simulink model "Bebop8_KF_filter"  (R2018a)
settings: Solver=VariableStepAuto  StartTime=0.0  StopTime=50  FixedStep=.04  MaxStep=1.00  MinStep=0.005  RelTol=10  AbsTol=10
values from neighbouring files (symbols this model uses):
  flightplan = [dist,0,height,deg2rad(090) ... (first row only)    [compare_cubic_spline_1.m]    (also in initialize_race_realtime.m = [dist+1,0,height,deg2rad(090); initialize_race_realtime_backup_cubic.m; plot_sim.m = [ 4.348, -0.278, height, deg2rad(  0); test_b_spline.m)
  FOV = 1.05    [initialize_race_realtime.m]    (also in initialize_race_realtime_backup_cubic.m)
  g = 9.81    [initialize_race_no_realtime.m]    (also in initialize_race_realtime.m; initialize_race_realtime_backup_cubic.m; moving_average_rls_own.m = P(i-1)*meas*(lambda+meas*P(i-1)*meas)^-1)
  gate_size = 1.4    [initialize_race_realtime.m]    (also in initialize_race_realtime_backup_cubic.m)
  gates = sim_gates(:,:,1)    [eval_sim.m]    (also in initialize_race_realtime.m = [dist+1,0,height,deg2rad(110); initialize_race_realtime_backup_cubic.m = [dist,0,height,deg2rad(110); plot_sim.m)
  I = [1 0 0 ... (first row only)    [Bebop_sim_init.m]    (also in initialize_race_no_realtime.m; initialize_race_realtime.m; initialize_race_realtime_backup_cubic.m; moving_averge_rls_download.m = ones(1,N))
  init_std_dev = [1.0*ones(1,3),deg2rad(30)]    [initialize_race_realtime.m]    (also in initialize_race_realtime_backup_cubic.m)
  m = 0.68    [calc_plot_spline.m]    (also in calc_spline.m; compare_cubic_spline_1.m = vpasolve(e,r); compare_cubic_spline_2.m = r/3*(-sin(dp)+sqrt(sin(dp)^2-6*cos(dp)+6)); initialize_race_no_realtime.m = 2)
  max_rot_Z = (90)*pi/180    (= 1.57079632679)    [Bebop_sim_init.m]    (also in initialize_race_no_realtime.m = 1.0471975512; initialize_race_realtime.m = 1.0471975512; initialize_race_realtime_backup_cubic.m; run_batch1.m = list_agility(idx_agility)*max_rot_Z)
  max_theta_X = (40)*pi/180    (= 0.698131700798)    [Bebop_sim_init.m]    (also in initialize_race_no_realtime.m = 0.13962634016; initialize_race_realtime.m = 1.308996939; initialize_race_realtime_backup_cubic.m = 1.308996939; run_batch1.m = list_agility(idx_agility)*max_theta_X)
  max_theta_Y = (40)*pi/180    (= 0.698131700798)    [Bebop_sim_init.m]    (also in initialize_race_no_realtime.m = 0.13962634016; initialize_race_realtime.m = 1.308996939; initialize_race_realtime_backup_cubic.m = 1.308996939; run_batch1.m = list_agility(idx_agility)*max_theta_Y)
  max_v_Z = .5    (= 0.5)    [Bebop_sim_init.m]    (also in initialize_race_no_realtime.m = 1; initialize_race_realtime.m = 2; initialize_race_realtime_backup_cubic.m = 3; run_batch1.m = list_agility(idx_agility)*max_v_Z)
  max_vel = 1.0    (= 1)    [initialize_race_realtime.m]    (also in initialize_race_realtime_backup_cubic.m = 1.5; run_batch1.m = list_speed(idx_speed); run_batch2.m = list_speed(idx_speed); run_batch3.m = list_speed(idx_speed))
  spline_init = [P0;P1;P2;P3]    [initialize_race_realtime.m]
  std_dev_factor = 1.0    (= 1)    [initialize_race_realtime.m]
  std_dev_switch = std_dev_factor/5    (= 0.2)    [initialize_race_realtime.m]
undefined symbols (not defined in the file or in its folder): fspecial, gray, Rec, SDTV
libraries: simulink x11, sharedtransform x11, visiontextngfix x7, visionanalysis x7, visiontransforms x3, aerolibactuator x2, aerolibutil x2, visionstatistics x2, visionconversions x2, shared6dof x1, vrlib x1, visionsinks x1
(part 3 of 4)

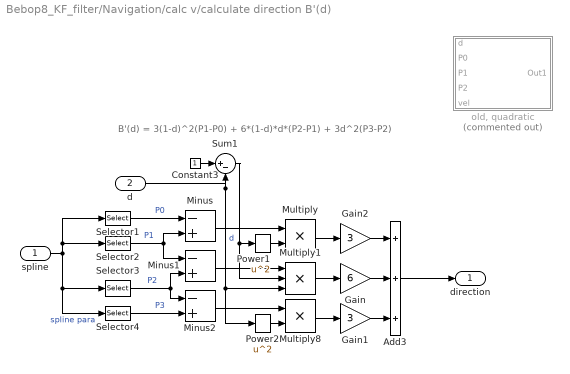
== system Bebop8_KF_filter/Navigation/calc v/calculate direction B'(d) ==
  note: B'(d) = 3(1-d)^2(P1-P0) + 6*(1-d)*d*(P2-P1) + 3d^2(P3-P2)
  spline : Inport
  d : Inport  Port=2
  Add3 : Sum  Inputs=+++
  Constant3 : Constant
  Gain : Gain  Gain=6
  Gain1 : Gain  Gain=3
  Gain2 : Gain  Gain=3
  Minus : Sum  Inputs=-+
  Minus1 : Sum  Inputs=-+
  Minus2 : Sum  Inputs=-+
  Multiply : Product
  Multiply1 : Product  Inputs=3
  Multiply8 : Product
  Power1 : Math  Operator=square  SaturateOnIntegerOverflow=on
  Power2 : Math  Operator=square  SaturateOnIntegerOverflow=on
  Selector1 : Selector  NumberOfDimensions=2  IndexMode=Zero-based  InputPortWidth=3  IndexOptions=Index vector (dialog),Select all  Indices=0,[0 1 2]  OutputSizes=1,1
  Selector2 : Selector  NumberOfDimensions=2  IndexMode=Zero-based  InputPortWidth=3  IndexOptions=Index vector (dialog),Select all  Indices=1,[0 1 2]  OutputSizes=1,1
  Selector3 : Selector  NumberOfDimensions=2  IndexMode=Zero-based  InputPortWidth=3  IndexOptions=Index vector (dialog),Select all  Indices=2,[0 1 2]  OutputSizes=1,1
  Selector4 : Selector  NumberOfDimensions=2  IndexMode=Zero-based  InputPortWidth=3  IndexOptions=Index vector (dialog),Select all  Indices=3,[0 1 2]  OutputSizes=1,1
  Sum1 : Sum  Inputs=|+-
  "old, quadratic" : Subsystem  Commented=on
  direction : Outport
  wires:
  Sum1/1 -> Multiply1/2, Power1/1
  Minus1/1 -> Multiply1/1
  Minus/1 -> Multiply/1
  Gain/1 -> Add3/2
  Gain1/1 -> Add3/3
  Multiply1/1 -> Gain/1
  Minus2/1 -> Multiply8/1
  Constant3/1 -> Sum1/1
  Multiply/1 -> Gain2/1
  Multiply8/1 -> Gain1/1
  Power2/1 -> Multiply8/2
  Power1/1 -> Multiply/2
  d/1 -> Sum1/2, Power2/1, Multiply1/3  "d"
  Gain2/1 -> Add3/1
  Add3/1 -> direction/1
  Selector1/1 -> Minus/1  "P0"
  Selector3/1 -> Minus2/1, Minus1/2  "P2"
  spline/1 -> Selector2/1, Selector1/1, Selector4/1, Selector3/1  "spline para"
  Selector2/1 -> Minus1/1, Minus/2  "P1"
  Selector4/1 -> Minus2/2  "P3"

== system Bebop8_KF_filter/Navigation/calc v/min spd ==
  In1 : Inport
  Abs : Abs
  Add : Sum  Inputs=+-
  Constant : Constant  Value=0.01
  Constant1 : Constant  Value=0.5
  Minus : Sum  Inputs=+-
  Multiply : Product
  Saturation : Saturate  UpperLimit=0  LowerLimit=-1
  Scope : Scope  NumInputPorts=7
  Sign : Signum
  Sign1 : Signum
  Sum : Sum  Inputs=|++
  Out1 : Outport
  wires:
  In1/1 -> Scope/1, Add/1, Sign/1, Abs/1
  Abs/1 -> Minus/1
  Constant/1 -> Minus/2
  Minus/1 -> Scope/4, Saturation/1
  Saturation/1 -> Scope/5, Multiply/1
  Sum/1 -> Sign1/1
  Multiply/1 -> Scope/2, Add/2
  Add/1 -> Scope/3, Out1/1
  Constant1/1 -> Sum/2
  Sign1/1 -> Multiply/2
  Sign/1 -> Sum/1

== system Bebop8_KF_filter/Navigation/calculate desired/If Action Subsystem ==
  In1 : Inport
  Action Port : ActionPort  ActionType=then
  Out1 : Outport
  wires:
  In1/1 -> Out1/1

== system Bebop8_KF_filter/Navigation/calculate desired/If Action Subsystem1 ==
  In1 : Inport
  Action Port : ActionPort  ActionType=else
  Out1 : Outport
  wires:
  In1/1 -> Out1/1

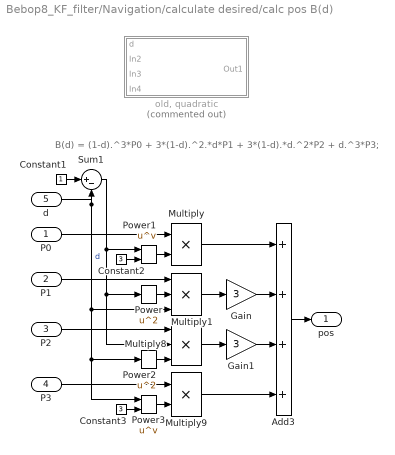
== system Bebop8_KF_filter/Navigation/calculate desired/calc pos B(d) ==
  note: B(d) = (1-d).^3*P0 + 3*(1-d).^2.*d*P1 + 3*(1-d).*d.^2*P2 + d.^3*P3;
  P0 : Inport
  P1 : Inport  Port=2
  P2 : Inport  Port=3
  P3 : Inport  Port=4
  d : Inport  Port=5
  Add3 : Sum  Inputs=++++
  Constant1 : Constant
  Constant2 : Constant  Value=3
  Constant3 : Constant  Value=3
  Gain : Gain  Gain=3
  Gain1 : Gain  Gain=3
  Multiply : Product
  Multiply1 : Product  Inputs=3
  Multiply8 : Product  Inputs=3
  Multiply9 : Product
  Power : Math  Operator=square  SaturateOnIntegerOverflow=on
  Power1 : Math  Operator=pow  SaturateOnIntegerOverflow=on
  Power2 : Math  Operator=square  SaturateOnIntegerOverflow=on
  Power3 : Math  Operator=pow  SaturateOnIntegerOverflow=on
  Sum1 : Sum  Inputs=|+-
  "old, quadratic" : Subsystem  Commented=on
  pos : Outport
  wires:
  Gain/1 -> Add3/2
  Gain1/1 -> Add3/3
  P1/1 -> Multiply1/1
  P0/1 -> Multiply/1
  P2/1 -> Multiply8/1
  P3/1 -> Multiply9/1
  Multiply/1 -> Add3/1
  Multiply1/1 -> Gain/1
  Multiply8/1 -> Gain1/1
  Multiply9/1 -> Add3/4
  Add3/1 -> pos/1
  Constant1/1 -> Sum1/1
  d/1 -> Sum1/2, Multiply1/3, Power2/1, Power3/1  "d"
  Power/1 -> Multiply1/2
  Power1/1 -> Multiply/2
  Power2/1 -> Multiply8/3
  Power3/1 -> Multiply9/2
  Constant2/1 -> Power1/2
  Constant3/1 -> Power3/2
  Sum1/1 -> Multiply8/2, Power/1, Power1/1

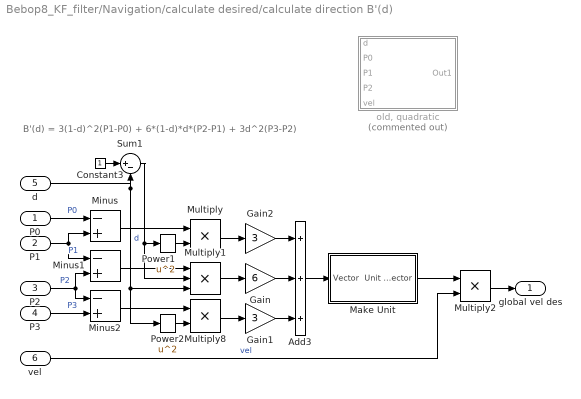
== system Bebop8_KF_filter/Navigation/calculate desired/calculate direction B'(d) ==
  note: B'(d) = 3(1-d)^2(P1-P0) + 6*(1-d)*d*(P2-P1) + 3d^2(P3-P2)
  P0 : Inport
  P1 : Inport  Port=2
  P2 : Inport  Port=3
  P3 : Inport  Port=4
  d : Inport  Port=5
  vel : Inport  Port=6
  Add3 : Sum  Inputs=+++
  Constant3 : Constant
  Gain : Gain  Gain=6
  Gain1 : Gain  Gain=3
  Gain2 : Gain  Gain=3
  Make Unit : Subsystem
  Minus : Sum  Inputs=-+
  Minus1 : Sum  Inputs=-+
  Minus2 : Sum  Inputs=-+
  Multiply : Product
  Multiply1 : Product  Inputs=3
  Multiply2 : Product
  Multiply8 : Product
  Power1 : Math  Operator=square  SaturateOnIntegerOverflow=on
  Power2 : Math  Operator=square  SaturateOnIntegerOverflow=on
  Sum1 : Sum  Inputs=|+-
  "old, quadratic" : Subsystem  Commented=on
  global vel des : Outport
  wires:
  Sum1/1 -> Multiply1/2, Power1/1
  Minus1/1 -> Multiply1/1
  Minus/1 -> Multiply/1
  Gain/1 -> Add3/2
  Gain1/1 -> Add3/3
  Multiply1/1 -> Gain/1
  Minus2/1 -> Multiply8/1
  Constant3/1 -> Sum1/1
  Multiply/1 -> Gain2/1
  Multiply8/1 -> Gain1/1
  Power2/1 -> Multiply8/2
  Power1/1 -> Multiply/2
  d/1 -> Sum1/2, Power2/1, Multiply1/3  "d"
  Gain2/1 -> Add3/1
  P0/1 -> Minus/1  "P0"
  P1/1 -> Minus/2, Minus1/1  "P1"
  P2/1 -> Minus1/2, Minus2/1  "P2"
  P3/1 -> Minus2/2  "P3"
  Multiply2/1 -> global vel des/1
  Add3/1 -> Make Unit/1(Vector)
  Make Unit/1(Unit Vector) -> Multiply2/1
  vel/1 -> Multiply2/2  "vel"

== system Bebop8_KF_filter/Navigation/calculate desired/min gate distance ==
  Constant2 : Constant  Value=gate_size
  Constant3 : Constant  Value=FOV
  Divide : Product  Inputs=*/
  Gain1 : Gain  Gain=0.5
  Gain2 : Gain  Gain=0.5
  Tan : Trigonometry  Operator=tan
  min gate dist : Outport
  wires:
  Constant3/1 -> Gain2/1
  Constant2/1 -> Gain1/1
  Gain1/1 -> Divide/1
  Gain2/1 -> Tan/1
  Divide/1 -> min gate dist/1  "min dist"
  Tan/1 -> Divide/2

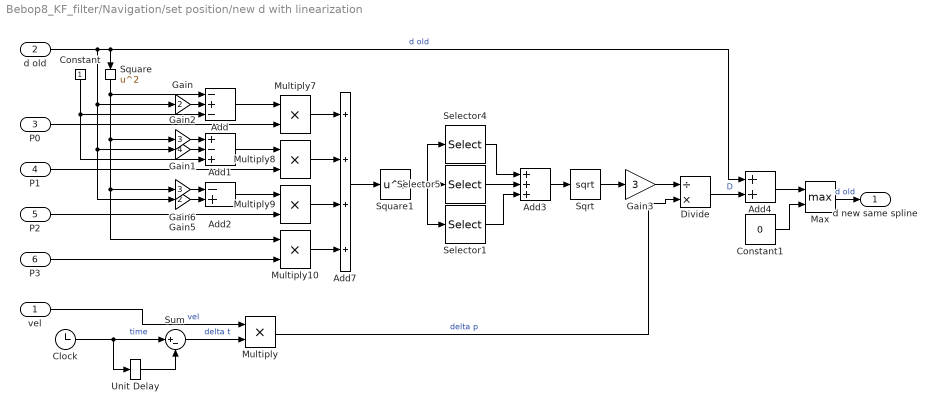
== system Bebop8_KF_filter/Navigation/set position/new d with linearization ==
  vel : Inport
  d old : Inport  Port=2
  P0 : Inport  Port=3
  P1 : Inport  Port=4
  P2 : Inport  Port=5
  P3 : Inport  Port=6
  Add : Sum  Inputs=-+-
  Add1 : Sum  Inputs=+-+
  Add2 : Sum  Inputs=-+
  Add3 : Sum  Inputs=+++
  Add4 : Sum
  Add7 : Sum  Inputs=++++
  Clock : Clock
  Constant : Constant
  Constant1 : Constant  Value=0
  Divide : Product  Inputs=/*
  Gain : Gain  Gain=2
  Gain1 : Gain  Gain=4
  Gain2 : Gain  Gain=3
  Gain3 : Gain  Gain=3
  Gain5 : Gain  Gain=2
  Gain6 : Gain  Gain=3
  Max : MinMax  Function=max  Inputs=2
  Multiply{,7..10} (5 alike) : Product
  Selector1 : Selector  IndexMode=Zero-based  InputPortWidth=3  IndexOptions=Index vector (dialog)  Indices=2  OutputSizes=1
  Selector4 : Selector  IndexMode=Zero-based  InputPortWidth=3  IndexOptions=Index vector (dialog)  Indices=0  OutputSizes=1
  Selector5 : Selector  IndexMode=Zero-based  InputPortWidth=3  IndexOptions=Index vector (dialog)  Indices=1  OutputSizes=1
  Sqrt : Sqrt  SaturateOnIntegerOverflow=on
  Square : Math  Operator=square  SaturateOnIntegerOverflow=on
  Square1 : Math  Operator=square  SaturateOnIntegerOverflow=on
  Sum : Sum  Inputs=|+-
  Unit Delay : UnitDelay  SampleTime=-1
  d new same spline : Outport
  wires:
  Add7/1 -> Square1/1
  Multiply8/1 -> Add7/2
  Multiply9/1 -> Add7/3
  Square/1 -> Multiply10/1, Gain6/1, Gain2/1, Add/1
  Gain/1 -> Add/2
  Constant/1 -> Add1/3, Add/3
  Gain2/1 -> Add1/1
  Gain1/1 -> Add1/2
  Gain6/1 -> Add2/1
  Gain5/1 -> Add2/2
  Multiply10/1 -> Add7/4
  Add2/1 -> Multiply9/1
  Add1/1 -> Multiply8/1
  Add/1 -> Multiply7/1
  Multiply7/1 -> Add7/1
  Selector5/1 -> Add3/2
  Multiply/1 -> Divide/2  "delta p"
  Gain3/1 -> Divide/1
  Divide/1 -> Add4/2  "D"
  Selector4/1 -> Add3/1
  Add3/1 -> Sqrt/1
  Square1/1 -> Selector1/1, Selector4/1, Selector5/1
  Sqrt/1 -> Gain3/1
  Selector1/1 -> Add3/3
  Sum/1 -> Multiply/2  "delta t"
  Unit Delay/1 -> Sum/2
  vel/1 -> Multiply/1  "vel"
  Clock/1 -> Unit Delay/1, Sum/1  "time"
  Add4/1 -> Max/1
  Constant1/1 -> Max/2
  P1/1 -> Multiply8/2
  P2/1 -> Multiply9/2
  P0/1 -> Multiply7/2
  Max/1 -> d new same spline/1  "d old"
  P3/1 -> Multiply10/2
  d old/1 -> Add4/1, Square/1, Gain/1, Gain5/1, Gain1/1  "d old"

== system Bebop8_KF_filter/Vision System/Harris corner detection/Harris Corners ==
  Threshold : Inport
  Corner Detection : visionanalysis/Corner Detection  method=Harris corner detection (Harris & Stephens)  factor=0.01  filter=fspecial('gaussian', [1 9], 3)  thrInten=0.1  thrAngle=157.5  output=Obsolete9b  outputInUse=Corner location  maxNum=5  thrMetric=0.01  neighborSize=[25 25]  isOutVarDim=on  accumMode=Binary point scaling  accumWordLength=32  accumFracLength=0  prodOutputMode=Binary point scaling  prodOutputWordLength=32  prodOutputFracLength=0  memoryMode=Binary point scaling  memoryWordLength=32  memoryFracLength=0  firstCoeffMode=Specify word length  firstCoeffWordLength=16  firstCoeffFracLength=17  roundingMode=Floor  overflowMode=off
      settings: SourceProductName=Computer Vision System Toolbox  SourceProductBaseCode=VP
  Gaussian Pyramid : visiontransforms/Gaussian Pyramid  Commented=on  operation=Expand  level=1  source=Specify via dialog  a=0.375  coef=fspecial('gaussian', [1 9], 3)  hiddenCoef=fspecial('gaussian', [1 9], 3)  firstCoeffMode=Specify word length  firstCoeffWordLength=16  firstCoeffFracLength=17  outputMode=Binary point scaling  outputWordLength=32  outputFracLength=10  prodOutputMode=Binary point scaling  prodOutputWordLength=32  prodOutputFracLength=10  roundingMode=Floor  overflowMode=off
      settings: SourceProductName=Computer Vision System Toolbox  SourceProductBaseCode=VP
  Video Viewer2 : VideoViewer  Commented=on  colormapValue=gray(256)  FigPos=[76 898 768 763]
  Corners : Outport
  wires:
  Threshold/1 -> Gaussian Pyramid/1, Corner Detection/1
  Gaussian Pyramid/1 -> Video Viewer2/1
  Corner Detection/1 -> Corners/1

== system Bebop8_KF_filter/Vision System/Harris corner detection/calculate corners ==
  In1 : Inport
  Action Port : ActionPort  PropagateVarSize=During execution  ActionType=then
  calculate corners : MATLAB Function  TreatAsAtomicUnit=on
  Out1 : Outport
  wires:
  In1/1 -> calculate corners/1(corners)
  calculate corners/1(corners_four) -> Out1/1

== system Bebop8_KF_filter/Control/Create Path Frame/Make X Vector/Make Unit ==
  Vector : Inport
  Multiply : Product
  Reciprocal Sqrt : Sqrt  Operator=rSqrt  SaturateOnIntegerOverflow=on
  Square : Math  Operator=square  SaturateOnIntegerOverflow=on
  Sum of Elements : Sum  Inputs=+
  Unit Vector : Outport
  wires:
  Reciprocal Sqrt/1 -> Multiply/1
  Vector/1 -> Square/1, Multiply/2
  Square/1 -> Sum of Elements/1
  Multiply/1 -> Unit Vector/1
  Sum of Elements/1 -> Reciprocal Sqrt/1

== system Bebop8_KF_filter/Control/Create Path Frame/Make Y Vector/Make Unit ==
  Vector : Inport
  Multiply : Product
  Reciprocal Sqrt : Sqrt  Operator=rSqrt  SaturateOnIntegerOverflow=on
  Square : Math  Operator=square  SaturateOnIntegerOverflow=on
  Sum of Elements : Sum  Inputs=+
  Unit Vector : Outport
  wires:
  Reciprocal Sqrt/1 -> Multiply/1
  Vector/1 -> Square/1, Multiply/2
  Square/1 -> Sum of Elements/1
  Multiply/1 -> Unit Vector/1
  Sum of Elements/1 -> Reciprocal Sqrt/1

== system Bebop8_KF_filter/Control/Create Path Frame/Make Z Vector/Make Unit ==
  Vector : Inport
  Multiply : Product
  Reciprocal Sqrt : Sqrt  Operator=rSqrt  SaturateOnIntegerOverflow=on
  Square : Math  Operator=square  SaturateOnIntegerOverflow=on
  Sum of Elements : Sum  Inputs=+
  Unit Vector : Outport
  wires:
  Reciprocal Sqrt/1 -> Multiply/1
  Vector/1 -> Square/1, Multiply/2
  Square/1 -> Sum of Elements/1
  Multiply/1 -> Unit Vector/1
  Sum of Elements/1 -> Reciprocal Sqrt/1

== system Bebop8_KF_filter/Navigation/calc v/Create Path Frame/Make X Vector ==
  Velocity Vector : Inport
  Make Unit : Subsystem
  Transpose : Math  Operator=transpose  SaturateOnIntegerOverflow=on
  X Vector : Outport
  wires:
  Velocity Vector/1 -> Make Unit/1(Vector)
  Make Unit/1(Unit Vector) -> Transpose/1
  Transpose/1 -> X Vector/1

== system Bebop8_KF_filter/Navigation/calc v/Create Path Frame/Make Y Vector ==
  Velocity Vector : Inport
  Constant : Constant  Value=0
  Demux : Demux  Outputs=3
  Gain : Gain  Gain=-1
  Make Unit : Subsystem
  Matrix Concatenate : Concatenate  NumInputs=3  Mode=Multidimensional array
  Terminator : Terminator
  Y Vector : Outport
  wires:
  Make Unit/1(Unit Vector) -> Y Vector/1
  Velocity Vector/1 -> Demux/1
  Demux/3 -> Terminator/1
  Demux/2 -> Gain/1
  Gain/1 -> Matrix Concatenate/1
  Demux/1 -> Matrix Concatenate/2
  Constant/1 -> Matrix Concatenate/3
  Matrix Concatenate/1 -> Make Unit/1(Vector)

== system Bebop8_KF_filter/Navigation/calc v/Create Path Frame/Make Z Vector ==
  Velocity Vector : Inport
  Add : Sum
  Demux : Demux  Outputs=3
  Gain : Gain  Gain=-1
  Gain1 : Gain  Gain=-1
  Make Unit : Subsystem
  Matrix Concatenate : Concatenate  NumInputs=3  Mode=Multidimensional array
  Multiply : Product
  Multiply1 : Product
  Square : Math  Operator=square  SaturateOnIntegerOverflow=on
  Square1 : Math  Operator=square  SaturateOnIntegerOverflow=on
  Z Vector : Outport
  wires:
  Make Unit/1(Unit Vector) -> Z Vector/1
  Velocity Vector/1 -> Demux/1
  Demux/3 -> Multiply/2, Multiply1/2
  Matrix Concatenate/1 -> Make Unit/1(Vector)
  Multiply/1 -> Gain/1
  Gain/1 -> Matrix Concatenate/1
  Demux/1 -> Square/1, Multiply/1
  Multiply1/1 -> Gain1/1
  Gain1/1 -> Matrix Concatenate/2
  Demux/2 -> Square1/1, Multiply1/1
  Add/1 -> Matrix Concatenate/3
  Square/1 -> Add/1
  Square1/1 -> Add/2

== system Bebop8_KF_filter/Navigation/calc v/calculate direction B'(d)/old, quadratic ==
  note: B'(d) = 2(1-d)(P1-P0) + 2d(P2-P1) = 2*(dP0-2dP1+dP2+P1-P0)
  d : Inport
  P0 : Inport  Port=2
  P1 : Inport  Port=3
  P2 : Inport  Port=4
  vel : Inport  Port=5
  Add1 : Sum  Commented=on  Inputs=+--++-
  Atan1 : Trigonometry  Commented=on  Operator=atan2
  Constant1 : Constant  Commented=on  Value=0
  Constant2 : Constant  Commented=on  Value=0
  Matrix Multiply : Product  Commented=on  Inputs=/*  Multiplication=Matrix(*)
  Product : Product  Commented=on
  Product1 : Product  Commented=on
  Product2 : Product  Commented=on
  Rotation Angles to Direction Cosine Matrix1 : sharedtransform/Rotation Angles to Direction Cosine Matrix  Commented=on  rotationOrder=ZYX  aMode=aMode
      settings: SourceProductBaseCode=AE
  Selector7 : Selector  Commented=on  IndexMode=Zero-based  InputPortWidth=3  IndexOptions=Index vector (dialog)  Indices=1  OutputSizes=1
  Selector8 : Selector  Commented=on  IndexMode=Zero-based  InputPortWidth=3  IndexOptions=Index vector (dialog)  Indices=0  OutputSizes=1
  Vector Concatenate : Concatenate  Commented=on  NumInputs=3
  Vector Concatenate1 : Concatenate  Commented=on  NumInputs=3
  Out1 : Outport
  wires:
  Product2/1 -> Add1/4
  P1/1 -> Add1/5, Product1/2
  Rotation Angles to Direction Cosine Matrix1/1 -> Matrix Multiply/1  "rot matrix"
  P2/1 -> Product2/2
  Add1/1 -> Selector8/1, Selector7/1
  Product/1 -> Add1/1
  P0/1 -> Add1/6, Product/2
  d/1 -> Product2/1, Product1/1, Product/1
  Constant1/1 -> Vector Concatenate/2, Vector Concatenate/3
  Vector Concatenate1/1 -> Matrix Multiply/2
  Product1/1 -> Add1/3, Add1/2
  Vector Concatenate/1 -> Rotation Angles to Direction Cosine Matrix1/1
  Selector7/1 -> Atan1/1
  vel/1 -> Vector Concatenate1/1
  Constant2/1 -> Vector Concatenate1/2, Vector Concatenate1/3
  Matrix Multiply/1 -> Out1/1
  Selector8/1 -> Atan1/2
  Atan1/1 -> Vector Concatenate/1  "yaw"

== system Bebop8_KF_filter/Navigation/calculate desired/calc pos B(d)/old, quadratic ==
  note: B(d) = (1-d)*u.*((1-d)*P0+d*P1)+d*u.*((1-d)*P1 + d*P2);
  d : Inport
  In2 : Inport  Port=2
  In3 : Inport  Port=3
  In4 : Inport  Port=4
  Add : Sum  Commented=on
  Add1 : Sum  Commented=on
  Add2 : Sum  Commented=on
  Constant : Constant  Commented=on
  Multiply{2..7} (6 alike) : Product  Commented=on
  Sum : Sum  Commented=on  Inputs=|+-
  Out1 : Outport
  wires:
  In4/1 -> Multiply5/1
  Constant/1 -> Sum/1
  Multiply7/1 -> Add2/2
  d/1 -> Multiply5/2, Multiply7/1, Multiply3/1, Sum/2
  Multiply3/1 -> Add/2
  Multiply5/1 -> Add1/2
  Multiply4/1 -> Add1/1
  Sum/1 -> Multiply4/2, Multiply6/2, Multiply2/1  "1-d"
  In3/1 -> Multiply4/1, Multiply3/2
  Multiply2/1 -> Add/1
  Add2/1 -> Out1/1
  Add1/1 -> Multiply7/2
  Multiply6/1 -> Add2/1
  In2/1 -> Multiply2/2
  Add/1 -> Multiply6/1

== system Bebop8_KF_filter/Navigation/calculate desired/calculate direction B'(d)/Make Unit ==
  Vector : Inport
  Multiply : Product
  Reciprocal Sqrt : Sqrt  Operator=rSqrt  SaturateOnIntegerOverflow=on
  Square : Math  Operator=square  SaturateOnIntegerOverflow=on
  Sum of Elements : Sum  Inputs=+
  Transpose : Math  Operator=transpose  SaturateOnIntegerOverflow=on
  Unit Vector : Outport
  wires:
  Reciprocal Sqrt/1 -> Multiply/1
  Vector/1 -> Square/1, Multiply/2
  Square/1 -> Sum of Elements/1
  Multiply/1 -> Transpose/1
  Sum of Elements/1 -> Reciprocal Sqrt/1
  Transpose/1 -> Unit Vector/1

== system Bebop8_KF_filter/Navigation/calculate desired/calculate direction B'(d)/old, quadratic ==
  note: B'(d) = 2(1-d)(P1-P0) + 2d(P2-P1) = 2*(dP0-2dP1+dP2+P1-P0)
  d : Inport
  P0 : Inport  Port=2
  P1 : Inport  Port=3
  P2 : Inport  Port=4
  vel : Inport  Port=5
  Add1 : Sum  Commented=on  Inputs=+--++-
  Atan1 : Trigonometry  Commented=on  Operator=atan2
  Constant1 : Constant  Commented=on  Value=0
  Constant2 : Constant  Commented=on  Value=0
  Matrix Multiply : Product  Commented=on  Inputs=/*  Multiplication=Matrix(*)
  Product : Product  Commented=on
  Product1 : Product  Commented=on
  Product2 : Product  Commented=on
  Rotation Angles to Direction Cosine Matrix1 : sharedtransform/Rotation Angles to Direction Cosine Matrix  Commented=on  rotationOrder=ZYX  aMode=aMode
      settings: SourceProductBaseCode=AE
  Selector7 : Selector  Commented=on  IndexMode=Zero-based  InputPortWidth=3  IndexOptions=Index vector (dialog)  Indices=1  OutputSizes=1
  Selector8 : Selector  Commented=on  IndexMode=Zero-based  InputPortWidth=3  IndexOptions=Index vector (dialog)  Indices=0  OutputSizes=1
  Vector Concatenate : Concatenate  Commented=on  NumInputs=3
  Vector Concatenate1 : Concatenate  Commented=on  NumInputs=3
  Out1 : Outport
  wires:
  Product2/1 -> Add1/4
  P1/1 -> Add1/5, Product1/2
  Rotation Angles to Direction Cosine Matrix1/1 -> Matrix Multiply/1  "rot matrix"
  P2/1 -> Product2/2
  Add1/1 -> Selector8/1, Selector7/1
  Product/1 -> Add1/1
  P0/1 -> Add1/6, Product/2
  d/1 -> Product2/1, Product1/1, Product/1
  Constant1/1 -> Vector Concatenate/2, Vector Concatenate/3
  Vector Concatenate1/1 -> Matrix Multiply/2
  Product1/1 -> Add1/3, Add1/2
  Vector Concatenate/1 -> Rotation Angles to Direction Cosine Matrix1/1
  Selector7/1 -> Atan1/1
  vel/1 -> Vector Concatenate1/1
  Constant2/1 -> Vector Concatenate1/2, Vector Concatenate1/3
  Matrix Multiply/1 -> Out1/1
  Selector8/1 -> Atan1/2
  Atan1/1 -> Vector Concatenate/1  "yaw"

== system Bebop8_KF_filter/Navigation/calc v/Create Path Frame/Make X Vector/Make Unit ==
  Vector : Inport
  Multiply : Product
  Reciprocal Sqrt : Sqrt  Operator=rSqrt  SaturateOnIntegerOverflow=on
  Square : Math  Operator=square  SaturateOnIntegerOverflow=on
  Sum of Elements : Sum  Inputs=+
  Unit Vector : Outport
  wires:
  Reciprocal Sqrt/1 -> Multiply/1
  Vector/1 -> Square/1, Multiply/2
  Square/1 -> Sum of Elements/1
  Multiply/1 -> Unit Vector/1
  Sum of Elements/1 -> Reciprocal Sqrt/1

== system Bebop8_KF_filter/Navigation/calc v/Create Path Frame/Make Y Vector/Make Unit ==
  Vector : Inport
  Multiply : Product
  Reciprocal Sqrt : Sqrt  Operator=rSqrt  SaturateOnIntegerOverflow=on
  Square : Math  Operator=square  SaturateOnIntegerOverflow=on
  Sum of Elements : Sum  Inputs=+
  Unit Vector : Outport
  wires:
  Reciprocal Sqrt/1 -> Multiply/1
  Vector/1 -> Square/1, Multiply/2
  Square/1 -> Sum of Elements/1
  Multiply/1 -> Unit Vector/1
  Sum of Elements/1 -> Reciprocal Sqrt/1

== system Bebop8_KF_filter/Navigation/calc v/Create Path Frame/Make Z Vector/Make Unit ==
  Vector : Inport
  Multiply : Product
  Reciprocal Sqrt : Sqrt  Operator=rSqrt  SaturateOnIntegerOverflow=on
  Square : Math  Operator=square  SaturateOnIntegerOverflow=on
  Sum of Elements : Sum  Inputs=+
  Unit Vector : Outport
  wires:
  Reciprocal Sqrt/1 -> Multiply/1
  Vector/1 -> Square/1, Multiply/2
  Square/1 -> Sum of Elements/1
  Multiply/1 -> Unit Vector/1
  Sum of Elements/1 -> Reciprocal Sqrt/1

== matlab function Bebop8_KF_filter/Vision System/Harris corner detection/calculate corners/calculate corners ==
  data: corners_four output; corners input
function corners_four = calculate_corners(corners)
    
    
    %% get bounding box
    corners = double(corners);
    box=[0,0,0,0];
    box(1) = min(corners(:,1));
    box(2) = max(corners(:,1));
    box(3) = min(corners(:,2));
    box(4) = max(corners(:,2));
    
    corners_box = ([box(1), box(3);
                    box(2), box(3);
                    box(1), box(4);
                    box(2), box(4)]);
                
    corners_four = int32(zeros(4,2));
                
    for m = 1:4
        box = corners_box(m,:);
        multi_box = ones(size(corners,1),1) * box;
        diff = multi_box - corners;
        dist = diff(:,1).^2 + diff(:,2).^2;
        [~,i] = min(dist);
        corners_four(m,:) = corners(i,:);
        corners(i,:)=[];
    end
    
end

== matlab function Bebop8_KF_filter/Navigation/select d ==
  data: d_old input; d_old output; std_dev input
function d_old = select_d(d_old, std_dev)

std_dev_factor = 1.0;
std_dev_switch = std_dev_factor/5;

std_dev_radius = std_dev_factor*max(std_dev.*[1;1;1;1/(30*pi/180)]);
std_dev_radius = min(1,std_dev_radius);

if std_dev_radius > std_dev_switch
    d_old = 0;
end

== matlab function Bebop8_KF_filter/Initialize/reset_plot ==
function reset_plot()
coder.extrinsic('quiver3')
coder.extrinsic('legend')
close all;
figure('units','normalized','outerposition',[0 0 0.5 1])
hold on
grid on
axis equal

legends=zeros(12,1);
legends(1)=plot3(0,0,-100,'m.','MarkerSize',7);
legends(2)=plot3(0,0,-100,'k.','MarkerSize',5);
legends(3)=quiver3(0,0,-100,0,0,0,0,'c','MaxHeadSize',1,'LineWidth',2);
legends(4)=quiver3(0,0,-100,0,0,0,0,'r','MaxHeadSize',1,'LineWidth',2);
legends(5)=plot3(0,0,-100,':','Color',[1,0.7,0],'LineWidth',2);
legends(6)=plot3(0,0,-100,'kx-','LineWidth',1.2,'MarkerIndices',1,'MarkerSize',10);
legends(7)=plot3(0,0,-100,'r--','LineWidth',1.5);
legends(8)=plot3(0,0,-100,'g--','LineWidth',1.5);
legends(9)=plot3(0,0,-100,'b--','LineWidth',1.5);
legends(10)=plot3(0,0,-100,'b+-','LineWidth',1.2,'MarkerIndices',1,'MarkerSize',10);
legends(11)=quiver3(0,0,-100,0,0,0,0,'b','MaxHeadSize',1,'LineWidth',2);
legends(12)=plot3(0,0,-100,':r','LineWidth',1);
legend(legends(1:12),'flown track','ground track','inactive WP +ori','active WP +ori','spline','drone pos+vel','drone x','drone y','drone z','des pos+vel','measured WP','std dev (x,y,th)','Location','eastoutside','AutoUpdate','off')

for i=1:25
    plot3(0,0,-100,'.')
end

% axis([-5,5,-5,5,-2,2])
axis([-5,5,-5,5,0,4])
% axis([1,4,-2,2,0,4])
%view(-20,40) % 3D view
view(-90,90) % top view
%view(-90,0) % front view
xlabel('x')
ylabel('y')
zlabel('z')

== matlab function Bebop8_KF_filter/conv/global2strange drone/MATLAB Function ==
  data: euler input; axang_strange output
function axang_strange = fcn(euler)
m1=zeros(3,3);
m1 = eul2rotm([euler(3),euler(2),euler(1)]);
m2 = eul2rotm([-pi/2, 0, pi/2]);

axang_strange = rotm2axang(m1*m2);

== matlab function Bebop8_KF_filter/Vision System/Harris corner detection/calculate_PnP ==
  data: tVec output; corners input; size input; rMat output
function [tVec, rMat] = calculate_PnP(corners, size)
    tVec=zeros(1,3);
    rMat=zeros(3,3);
    
    Resolution = 1.5*[320, 200];
    vertFOV = 1.05;
    f = 0.5*Resolution(2)/tan(0.5*vertFOV);
    IntrinsicMatrix = [f, 0, 0;
        0, f, 0;
        Resolution/2, 1];
    cameraParams = cameraParameters('IntrinsicMatrix',IntrinsicMatrix); 
    
    %% calculate extrinsics
    worldPoints = size/2*[1 1;
        1 -1;
        -1 1;
        -1 -1];
    
    corners=double(corners);
    if corners == zeros(4,2)
        disp('no corners')
        return
    end
    
    angles = zeros(6,1);
    k = 1;
    for m=1:3
        for n=m+1:4
            angles(k)=atan2(corners(m,2)-corners(n,2),corners(m,1)-corners(n,1));
            k = k+1;            
        end
    end
    
%     angles(angles<=0) = angles(angles<=0)+pi;
%     
%     a = zeros(2,1);
%     a = hist(angles,unique(angles));
%     if max(a)>2
%         disp('three occurences')
%         return
%     end
%     
%     
%     

    % check how much it resembles rectangle
    if abs(max(corners(:,1))-min(corners(:,1))) < 5
        disp('no rectangle 1')
        corners
        return
    elseif abs(max(corners(:,2))-min(corners(:,2))) < 5
        disp('no rectangle 2')
        corners
        return
    end
    
    angles = zeros(2,1);
    angles(1)=atan2(corners(1,2)-corners(4,2),corners(1,1)-corners(4,1));
    angles(2)=atan2(corners(2,2)-corners(3,2),corners(2,1)-corners(3,1));
    angles(angles<=0) = angles(angles<=0)+pi;
    
    if ~(isequal(unique(angles),sort(angles)))
        temp = corners(3,:);
        corners(3,:) = corners(4,:);
        corners(4,:) = temp;
    end
    
    angles(1)=atan2(corners(1,2)-corners(4,2),corners(1,1)-corners(4,1));
    angles(2)=atan2(corners(2,2)-corners(3,2),corners(2,1)-corners(3,1));
    angles(angles<=0) = angles(angles<=0)+pi;
    
    if ~(isequal(unique(angles),sort(angles)))
        disp('still bad after sort')
        corners
        return
    end    
        
    [rMat,tVec] = extrinsics(corners,worldPoints,cameraParams);
%     [orientation,location] = extrinsicsToCameraPose(rMat,tVec);
    
end

== matlab function Bebop8_KF_filter/Gate info/Yaw2Axang4/MATLAB Function1 ==
  data: axang output; q input
function axang = fcn(q)

axang = zeros(4,1);

angle = 2 * acos(q(1));
x = q(2) / sqrt(1-q(1)*q(1));
y = q(3) / sqrt(1-q(1)*q(1));
z = q(4) / sqrt(1-q(1)*q(1));

if all(isnan([x,y,z]))
    x = 1;
    y = 0;
    z = 0;
end

axang(1) = x;
axang(2) = y;
axang(3) = z;
axang(4) = angle;

== matlab function Bebop8_KF_filter/conv/global2strange drone/MATLAB Function1 ==
  data: axang output; q input
function axang = fcn(q)

axang = zeros(4,1);

angle = 2 * acos(q(1));
x = q(2) / sqrt(1-q(1)*q(1));
y = q(3) / sqrt(1-q(1)*q(1));
z = q(4) / sqrt(1-q(1)*q(1));

axang(1) = x;
axang(2) = y;
axang(3) = z;
axang(4) = angle;

== matlab function Bebop8_KF_filter/Plot ==
  data: inbus input
function plot3d(inbus)
%#codegen
coder.extrinsic('delete')
% coder.extrinsic('ellipsoid')
% coder.extrinsic('viscircles')
% coder.extrinsic('quiver3')
% coder.extrinsic('legend')
std_dev_factor = 1.0;

drone_vel = inbus.state.vel;
drone_pos = inbus.state.pos;
drone_ori = inbus.state.eul;
WP_curr_eul = inbus.WP_curr.eul;
WP_curr_pos = inbus.WP_curr.pos;
SP_des_vel = inbus.SP_des.vel;
SP_des_pos = inbus.SP_des.pos;
WP_idx = inbus.WP_all.idx + 1;
WP_list = inbus.WP_all.list;
effort = inbus.effort;
std_dev = inbus.std_dev;
current_spline = inbus.current_spline;

children = get(gca, 'children');
delete(children(1:16));

P0 = current_spline(1,:);
P1 = current_spline(2,:);
P2 = current_spline(3,:);
P3 = current_spline(4,:);

% flown track + ground track
plot3(drone_pos(1),drone_pos(2),drone_pos(3),'m.','MarkerSize',7); %1
% plot3(drone_pos(1),drone_pos(2),0,'k.','MarkerSize',5); %2

% all WPts + ori
% quiver3 (WP_list(:,1),WP_list(:,2),WP_list(:,3),cos(WP_list(:,4)),sin(WP_list(:,4)),zeros(4,1),0,'c','MaxHeadSize',1,'LineWidth',2); %3
for i = 1:4
    if i == WP_idx
        continue
    end
    plot3(WP_list(i,1)+[0 cos(WP_list(i,4))],WP_list(i,2)+[0 sin(WP_list(i,4))],WP_list(i,3)+[0 0],'c+-','LineWidth',2,'MarkerIndices',2); %3
end

% WP average pos+ori
% quiver3(P2(1),P2(2),P2(3),cos(P2(4)),sin(P2(4)),0,0,'r','MaxHeadSize',1,'LineWidth',2); %4
plot3(WP_list(WP_idx,1)+[0 cos(WP_list(WP_idx,4))],WP_list(WP_idx,2)+[0 sin(WP_list(WP_idx,4))],WP_list(WP_idx,3)+[0 0],'r+-','LineWidth',2,'MarkerIndices',2); %3

% spline
d = (0:0.05:1)';
% u = ones(1,3);
% spline_pos_quad = (1-d)*u.*((1-d)*P0+d*P1)+d*u.*((1-d)*P1 + d*P2);
spline_pos_cubic = (1-d).^3*P0 + 3*(1-d).^2.*d*P1 + 3*(1-d).*d.^2*P2 + d.^3*P3;
plot3(spline_pos_cubic(:,1),spline_pos_cubic(:,2),spline_pos_cubic(:,3),':','Color',[1,0.7,0],'LineWidth',2); %5
plot3(current_spline(:,1),current_spline(:,2),current_spline(:,3),'og')

% drone pos+vel
plot3(drone_pos(1)+[0 drone_vel(1)],drone_pos(2)+[0 drone_vel(2)],drone_pos(3)+[0 drone_vel(3)],'kx-','LineWidth',1.2,'MarkerIndices',1,'MarkerSize',10); %6

% drone ori
gRb = eul2rotm([drone_ori(3),drone_ori(2),drone_ori(1)]);
length = 1;
x_bebop = gRb*[length;0;0];
y_bebop = gRb*[0;length;0];
z_bebop = gRb*[0;0;length];
plot3(drone_pos(1)+x_bebop(1)*[0.2 1],drone_pos(2)+x_bebop(2)*[0.2 1],drone_pos(3)+x_bebop(3)*[0.2 1],'r:','LineWidth',1.5); %7
plot3(drone_pos(1)+y_bebop(1)*[0.2 1],drone_pos(2)+y_bebop(2)*[0.2 1],drone_pos(3)+y_bebop(3)*[0.2 1],'g:','LineWidth',1.5); %8
plot3(drone_pos(1)+z_bebop(1)*[0.2 1],drone_pos(2)+z_bebop(2)*[0.2 1],drone_pos(3)+z_bebop(3)*[0.2 1],'b:','LineWidth',1.5); %9

% nav pt pos+vel, (yaw)
plot3(SP_des_pos(1)+[0 SP_des_vel(1)],SP_des_pos(2)+[0 SP_des_vel(2)],SP_des_pos(3)+[0 SP_des_vel(3)],'b+-','LineWidth',1.2,'MarkerIndices',1,'MarkerSize',10); %10
% plot3(WP_pos(1)+[0 0.5*cos(WP_yaw)],WP_pos(2)+[0 0.5*sin(WP_yaw)],WP_pos(3)+[0 0],'r-','LineWidth',1)

% WP current pos + ori
if isequal(WP_curr_eul, zeros(1,3)) || isequal(WP_curr_eul, zeros(3,1))
    % no gate info
    WP_curr_pos = [0,0,-100]';
    x_gate = WP_curr_eul;
else   
    gate_rot = eul2rotm(WP_curr_eul');
    x_gate = gate_rot(:,1);
end
% quiver3(gate_pos_global(1),gate_pos_global(2),gate_pos_global(3),x_gate(1),x_gate(2),x_gate(3),0,'b','MaxHeadSize',1,'LineWidth',2); %11
plot3(WP_curr_pos(1)+[0 x_gate(1)],WP_curr_pos(2)+[0 x_gate(2)],WP_curr_pos(3)+[0 x_gate(3)],'b+-','LineWidth',2,'MarkerIndices',2); %3

% effort
effort_gl = ones(4,1) * drone_pos' + [zeros(1,3);
    x_bebop'*effort(1);
    y_bebop'*effort(2);
    z_bebop'*effort(3)];
plot3(effort_gl([1 2],1),effort_gl([1 2],2),effort_gl([1 2],3),'r-','LineWidth',2);
plot3(effort_gl([1 3],1),effort_gl([1 3],2),effort_gl([1 3],3),'g-','LineWidth',2);
plot3(effort_gl([1 4],1),effort_gl([1 4],2),effort_gl([1 4],3),'b-','LineWidth',2);

% WP std dev
std_dev = std_dev*std_dev_factor;
r=linspace(WP_list(WP_idx,4),WP_list(WP_idx,4)+2*pi,4*4*2+1)';
angle_std_dev_length=0.6;
angle_std_dev_draw = [WP_list(WP_idx,1:3);
    WP_list(WP_idx,1:3)+angle_std_dev_length*[cos(WP_list(WP_idx,4)+std_dev(4)), sin(WP_list(WP_idx,4)+std_dev(4)), 0];
    WP_list(WP_idx,1:3);
    WP_list(WP_idx,1:3)+angle_std_dev_length*[cos(WP_list(WP_idx,4)-std_dev(4)), sin(WP_list(WP_idx,4)-std_dev(4)), 0];
    WP_list(WP_idx,1:3);
    WP_list(WP_idx,1)+std_dev(1)*cos(atan2(std_dev(1)/std_dev(2)*sin(r),cos(r))), WP_list(WP_idx,2)+std_dev(2)*sin(atan2(std_dev(1)/std_dev(2)*sin(r),cos(r))), WP_list(WP_idx,3)+0*r];
d = angle_std_dev_draw;
plot3(d(:,1),d(:,2),d(:,3),':r','LineWidth',1); %12
% [ellx,elly,ellz] = ellipsoid(P2(1),P2(2),P2(3),3*std_dev(1),3*std_dev(2),3*std_dev(3),20);
% surf(ellx,elly,ellz,ellz,'FaceAlpha',0.5)

% legend
% legend(legends(1:12),'flown track','ground track','inactive WP +ori','active WP +ori','spline','drone pos+vel','drone x','drone y','drone z','des pos+vel','measured WP','std dev (x,y,th)','Location','eastoutside')

== matlab function Bebop8_KF_filter/Guidance/select_WP ==
  data: WP_average output; WP_list input; WP_last output; WP_idx input
function [WP_average, WP_last] = select_WP(WP_list, WP_idx)
    WP_average=zeros(1,4);
    WP_last=zeros(1,4);
    
    WP_average = WP_list(WP_idx+1,:);
    if WP_idx > 0
        WP_last = WP_list(WP_idx,:);
    else
        WP_last = WP_list(end,:);
    end
end

== matlab function Bebop8_KF_filter/Guidance/create_spline ==
  data: old_spline input; WP_average input; current_spline output size=[4,3]; std_dev input; d_old_raw input
function current_spline = create_spline(old_spline, WP_average, std_dev, d_old_raw)
% current_spline = zeros(3,3); %4x3
std_dev_factor = 1.0;
std_dev_switch = std_dev_factor/5;

std_dev_radius = std_dev_factor*max(std_dev.*[1;1;1;1/(30*pi/180)]);
std_dev_radius = min(1,std_dev_radius);
HFOV = 1.05*320/200;

d_old = mod(d_old_raw,1);

SP_pos = (1-d_old_raw)^3*old_spline(1,:) + 3*(1-d_old_raw)^2*d_old_raw*old_spline(2,:) + 3*(1-d_old_raw)*d_old_raw^2*old_spline(3,:) + d_old_raw^3*old_spline(4,:);
SP_vel = 3*(1-d_old_raw)^2*(old_spline(2,:)-old_spline(1,:)) + 6*(1-d_old_raw)*d_old_raw*(old_spline(3,:)-old_spline(2,:)) + 3*d_old_raw^2*(old_spline(4,:)-old_spline(3,:));
SP_vel0= old_spline(2,:)-old_spline(1,:);

WP_gate = WP_average;
offset1 = (std_dev_radius+0.7)/sin(HFOV/2);
if std_dev_radius > std_dev_switch
    disp('up')
    WP1 = [SP_pos, atan2(SP_vel(2),SP_vel(1))];
    WP2 = WP_gate(1:4);
    WP2(1:3) = WP_gate(1:3) - offset1*[cos(WP2(4)) sin(WP2(4)) 0];
else
    disp('down')
    WP1 = [old_spline(1,:), atan2(SP_vel0(2),SP_vel0(1))];
    WP2 = WP_gate(1:4);
end
    

%% position cubic spline start at supposed pos, random values
% % B(d) = (1-d)^3*P0 + 3(1-d)^2*d*P1 + 3(1-d)*d^2*P2 + d^3*P3
% % B'(d) = 3(1-d)^2(P1-P0) + 6*(1-d)*d*(P2-P1) + 3d^2(P3-P2)
% 
% % B(0) = P0
% % B(1) = P3
% 
% P0 = WP1(1:3);
% P3 = WP2(1:3);
% hdg0 = WP1(4);
% hdg3 = WP2(4);
% 
% m = norm(P0-P3)-1;
% m = max(0.01,m);+
% P1 = [P0(1)+m*cos(hdg0), P0(2)+m*sin(hdg0), P3(3)];
% 
% offset2 = (std_dev_factor+0.7)/sin(HFOV/2*0.999);
% P2 = WP_average(1:3) - (offset2+1*(offset2-offset1))*[cos(hdg3) sin(hdg3) 0];
%           
% % n = 3-norm(P0-WP_average(1:3));
% % n = max(0.001,n);
% % P2 = P3 - n*[cos(WP2(4)) sin(WP2(4)) 0];
% 
% current_spline = [P0; P1; P2; P3];

%% cube with m = n
% % B(d) = (1-d)^3*P0 + 3(1-d)^2*d*P1 + 3(1-d)*d^2*P2 + d^3*P3
% % B'(d) = 3(1-d)^2(P1-P0) + 6*(1-d)*d*(P2-P1) + 3d^2(P3-P2)
% 
% % B(0) = P0
% % B(1) = P3
% 
% P0 = WP1(1:3);
% P3 = WP2(1:3);
% hdg0 = WP1(4);
% hdg3 = WP2(4);
% 
% % g1: P0 + m*[cos(hdg0);sin(hdg0);0]
% % g2: P3 - n*[cos(hdg3);sin(hdg3);0]
% 
% % m*f(hdg0)+n*f(hdg3) +P0-P3 = 0
% % m*(f(hdg0)+f(hdg3)) +P0-P3 = 0
% 
% % m*(c0+c3)+P0(1)-P3(1)=0
% % m = (P3(1)-P0(1) )/(cos(hdg0)+cos(hdg3))
% 
% m = (P3(1)-P0(1) )/(cos(hdg0)+cos(hdg3));
% P1 = P0 + [m*cos(hdg0), m*sin(hdg0), 1*(P3(3)-P0(3))];
% P2 = P3 - [m*cos(hdg3), m*sin(hdg3), 0              ];
% 
% current_spline = [P0; P1; P2; P3];

%% cube without m=n
% % B(d) = (1-d)^3*P0 + 3(1-d)^2*d*P1 + 3(1-d)*d^2*P2 + d^3*P3
% % B'(d) = 3(1-d)^2(P1-P0) + 6*(1-d)*d*(P2-P1) + 3d^2(P3-P2)
% 
% % B(0) = P0
% % B(1) = P3
% 
% P0 = WP1(1:3);
% P3 = WP2(1:3);
% hdg0 = WP1(4);
% hdg3 = WP2(4);
% 
% % g1: P0 + m*[cos(hdg0);sin(hdg0);0]
% % g2: P3 - n*[cos(hdg3);sin(hdg3);0]
% 
% % m*cos(hdg0)+n*cos(hdg3) +P0(1)-P3(1) = 0
% % m*sin(hdg0)+n*sin(hdg3) +P0(2)-P3(2) = 0
% 
% A = [cos(hdg0) cos(hdg3);
%      sin(hdg0) sin(hdg3)];
% b = -[P0(1)-P3(1);
%     P0(2)-P3(2)];
% r = A\b;
% m = r(1);
% n = r(2);
% P1 = P0 + [m*cos(hdg0), m*sin(hdg0), 1*(P3(3)-P0(3))];
% P2 = P3 - [n*cos(hdg3), n*sin(hdg3), 0];
% 
% current_spline = [P0; P1; P2; P3];

%% cube, m and n from dist
% B(d) = (1-d)^3*P0 + 3(1-d)^2*d*P1 + 3(1-d)*d^2*P2 + d^3*P3
% B'(d) = 3(1-d)^2(P1-P0) + 6*(1-d)*d*(P2-P1) + 3d^2(P3-P2)

% B(0) = P0
% B(1) = P3

P0 = WP1(1:3);
P3 = WP2(1:3);
hdg0 = WP1(4);
hdg3 = WP2(4);

% dist_fly = norm(P0-P3);
% dist_nofly = norm(WP_gate(1:3)-P3);
% fact_nofly = max(0.25,sqrt(dist_nofly/2));
% 
% m = dist_fly/4*fact_nofly;
% n = dist_fly/4/fact_nofly;

l_F = norm(P0-P3);
l_TW = norm(WP_gate(1:3)-P3);

m = l_F*min(1/10+l_TW/10,1/2);
n = l_F*max(1-l_TW/2,1/10);

P1 = P0 + [m*cos(hdg0), m*sin(hdg0), 1*(P3(3)-P0(3))];
P2 = P3 - [n*cos(hdg3), n*sin(hdg3), 0];

current_spline = [P0; P1; P2; P3];
end

== matlab function Bebop8_KF_filter/Vision System/intersect lines ==
  data: index input; count input; thetas input; corners_output output; rhos input
function corners_output = intersect_lines(index,count,thetas,rhos)
% if angle diff is nmore than 45 deg
% then intersect
dist_thresh = 20;

index = index(1:count,:);
theta=thetas(index(:,1));
rho=rhos(index(:,2));

intersections = zeros(0,2);

for i=1:length(theta)-1
    for j=i+1:length(theta)
        angle_diff = abs(atan2(sin(theta(i)-theta(j)),cos(theta(i)-theta(j))));
        if angle_diff > 40*pi/180 && angle_diff < 140*pi/180
            % intersect lines
            % g1: r1*[cos(t1),sin(t1)] + m*[-sin(t1),cos(t1)]
            % g2: r2*[cos(t2),sin(t2)] + n*[-sin(t2),cos(t2)]
            % equal:
            % r1*cos(t1) - r2*cos(t2) + n*sin(t2) = m*sin(t1) (II in I)
            % r1*sin(t1) - r2*sin(t2) + m*cos(t1) = n*cos(t2)
            % 
            % r1*cos(t1) - r2*cos(t2) + (r1*sin(t1) - r2*sin(t2)))*sin(t2)/cos(t2) = m*(sin(t1) - cos(t1)*sin(t2)/cos(t2))
            ci = cos(theta(i));
            cj = cos(theta(j));
            si = sin(theta(i));
            sj = sin(theta(j));
            ri = rho(i);
            rj = rho(j);
            
            m = (ri*ci-rj*cj+(ri*si-rj*sj)*sj/cj)/(si-ci*sj/cj);
            intersection = ri*[ci,si] + m*[-si,ci];
            
            intersections = [intersections; intersection];
        end
    end    
end

% corners_output = int16(intersections);
% return

clusters = zeros(size(intersections,1),1);
cluster = 0;
corners = zeros(0,2);
votes = zeros(0,1);
while ~all(clusters)
    cluster = cluster+1;
    % find first unclustered and set as center
    s = find(~clusters,1);
    pos_m = intersections(s,:);
    vote_m = 1;
    % set this point as clustered
    clusters(s) = cluster;
    % find points belonging to this cluster until no more were found (and go_around becomes false)
    for i=1:size(intersections,1)
        if ~clusters(i)
            % go through all unclustered points and calculate distance to cluster center
            pos = intersections(i,:);
            distance = norm(pos-pos_m);
            if distance < dist_thresh
                % recalculate average and votes
                pos_m = (pos_m * vote_m + pos) / (vote_m + 1);
                vote_m = vote_m + 1;
                % set point as clustered
                clusters(i) = cluster;
            end
        end
    end
    % finished. add average to a list of clusters
    corners = [corners; pos_m];
    votes = [votes; vote_m];
end

while size(corners,1) > 4
    [~,i]=min(flipud(votes));
    i = size(corners,1) - i + 1;
    corners(i,:)=[];
    votes(i)=[];
end

corners_output = int16(zeros(4,2));
if size(corners,1) == 4
    box=[0,0,0,0];
    box(1) = min(corners(:,1));
    box(2) = max(corners(:,1));
    box(3) = min(corners(:,2));
    box(4) = max(corners(:,2));
    
    corners_box = ([box(1), box(3);
                    box(2), box(3);
                    box(1), box(4);
                    box(2), box(4)]);
           
    
    corners_sorted = zeros(4,2);
    for m = 1:4
        box = corners_box(m,:);
        multi_box = ones(size(corners,1),1) * box;
        diff = multi_box - corners;
        dist = diff(:,1).^2 + diff(:,2).^2;
        [~,i] = min(dist);
        corners_sorted(m,:) = corners(i,:);
        corners(i,:)=[];
    end
    corners_output = int16(corners_sorted);
end

== matlab function Bebop8_KF_filter/Vision System/calculate_PnP1 ==
  data: tVec output size=[1 3]; corners input; gate_size input; rMat output size=[3 3]; FOV input
function [tVec, rMat] = calculate_PnP(corners, gate_size, FOV)
    tVec=zeros(1,3);
    rMat=zeros(3,3);
    
    Resolution = 1.5*[320, 200];
    f = 0.5*Resolution(2)/tan(0.5*FOV);
    IntrinsicMatrix = [f, 0, 0;
        0, f, 0;
        Resolution/2, 1];
    cameraParams = cameraParameters('IntrinsicMatrix',IntrinsicMatrix); 
    
    %% calculate extrinsics
    worldPoints = gate_size/2*[1 1;
        1 -1;
        -1 1;
        -1 -1];
    
    corners=double(corners);

    if isempty(corners) || isequal(corners,int16(zeros(4,2)))
%         disp('PnP - no corners')
        return
    end
    
    
    angles = zeros(6,1);
    k = 1;
    for m=1:3
        for n=m+1:4
            angles(k)=atan2(corners(m,2)-corners(n,2),corners(m,1)-corners(n,1));
            k = k+1;            
        end
    end
        
    angles(angles<=0) = angles(angles<=0)+pi;
    angles=round(angles*100)/100;
    angles=[angles;-1];
     
    a = hist(angles,unique(angles));
    if max(a,[],2)>2
        disp('three occurences')
        return
    end
    
% 
%     % check how much it resembles rectangle
%     if abs(max(corners(:,1))-min(corners(:,1))) < 5
%         disp('no rectangle 1')
%         corners
%         return
%     elseif abs(max(corners(:,2))-min(corners(:,2))) < 5
%         disp('no rectangle 2')
%         corners
%         return
%     end
%     
%     angles = zeros(2,1);
%     angles(1)=atan2(corners(1,2)-corners(4,2),corners(1,1)-corners(4,1));
%     angles(2)=atan2(corners(2,2)-corners(3,2),corners(2,1)-corners(3,1));
%     angles(angles<=0) = angles(angles<=0)+pi;
%     
%     if ~(isequal(unique(angles),sort(angles)))
%         temp = corners(3,:);
%         corners(3,:) = corners(4,:);
%         corners(4,:) = temp;
%     end
%     
%     angles(1)=atan2(corners(1,2)-corners(4,2),corners(1,1)-corners(4,1));
%     angles(2)=atan2(corners(2,2)-corners(3,2),corners(2,1)-corners(3,1));
%     angles(angles<=0) = angles(angles<=0)+pi;
%     
%     if ~(isequal(unique(angles),sort(angles)))
%         disp('still bad after sort')
%         corners
%         return
%     end    
        
    [rMat,tVec] = extrinsics(corners,worldPoints,cameraParams);
%     [orientation,location] = extrinsicsToCameraPose(rMat,tVec);
    
end
